simulink model "PID_Controller_referenceModel"  (R2021b)
settings: Solver=FixedStepDiscrete  StartTime=0.0  StopTime=10.0  FixedStep=Ts  RelTol=1e-3
PreLoadFcn:
  | %load('Parameters.mat')
values from neighbouring files (symbols this model uses):
  Kd = 1    [Parameters.mat]
  Ki = 1    [Parameters.mat]
  Kp = 1    [Parameters.mat]
  Ts = 0.01    [Parameters.mat]
settings Model: Creator=vigne  LastModifiedBy=vigne
settings DataIOCC: SaveOutput=off  SaveTime=off
settings OptimizationCC: DefaultParameterBehavior=Inlined  EnhancedBackFolding=on  PassReuseOutputArgsAs=Individual arguments  ZeroExternalMemoryAtStartup=off  ZeroInternalMemoryAtStartup=off  OptimizeBlockOrder=speed  DifferentSizesBufferReuse=on  OptimizationCustomize=off  EfficientTunableParamExpr=on
settings DebuggingCC: ParameterTunabilityLossMsg=error
settings SFSimCC: MATLABDynamicMemAlloc=off
settings RTWCC: Description=Embedded Coder  SystemTargetFile=ert.tlc  GenCodeOnly=on  TemplateMakefile=ert_default_tmf
settings CodeAppCC: ForceParamTrailComments=on  IgnoreCustomStorageClasses=off  OperatorAnnotations=on  SimulinkDataObjDesc=on  SFDataObjDesc=on  InsertBlockDesc=on
settings ERTTargetCC: TargetLangStandard=C99 (ISO)  GenerateSampleERTMain=on  InlinedParameterPlacement=NonHierarchical  ERTCustomFileTemplate=example_file_process.tlc

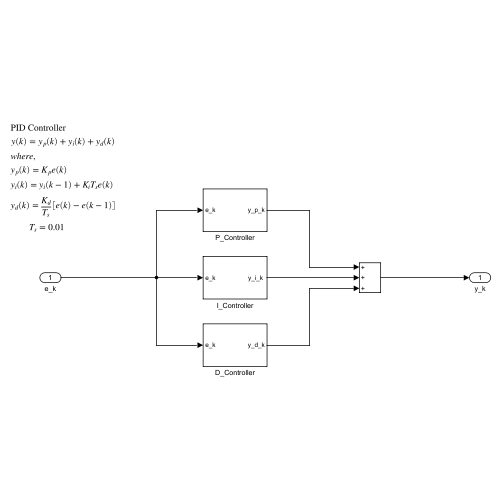
[thumbnail: Simulink's stored preview of the top-level diagram]
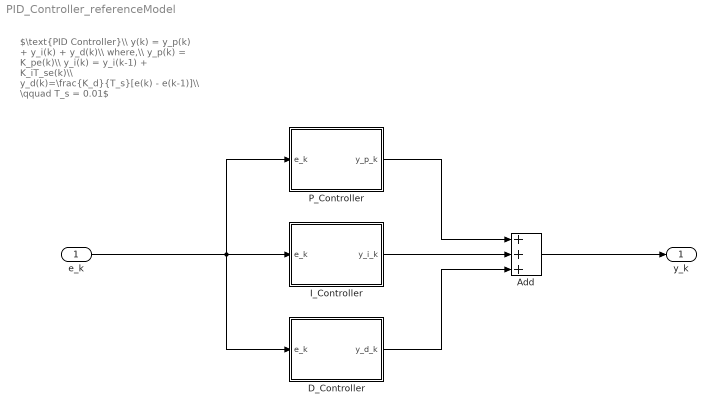
== system PID_Controller_referenceModel ==
  note: $\text{PID Controller}\\ y(k) = y_p(k) + y_i(k) + y_d(k)\\ where,\\ y_p(k) = K_pe(k)\\ y_i(k) = y_i(k-1) + K_iT_se(k)\\ y_d(k)=\frac{K_d}{T_s}[e(k) - e(k-1)]\\ \qquad T_s = 0.01$
  e_k : Inport  OutDataTypeStr=double  PortDimensions=1  SampleTime=Ts
  Add : Sum  Inputs=+++
  D_Controller : Subsystem
  I_Controller : Subsystem
  P_Controller : Subsystem
  y_k : Outport  OutDataTypeStr=double  PortDimensions=1  SampleTime=Ts
  wires:
  D_Controller/1(y_d_k) -> Add/3
  Add/1 -> y_k/1
  e_k/1 -> I_Controller/1(e_k), D_Controller/1(e_k), P_Controller/1(e_k)
  I_Controller/1("y_i_k ") -> Add/2
  P_Controller/1(y_p_k) -> Add/1

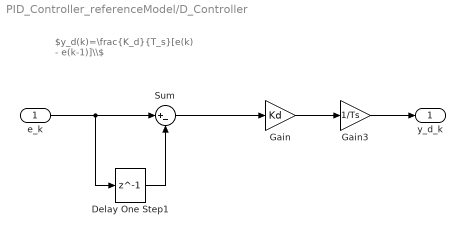
== system PID_Controller_referenceModel/D_Controller ==
  note: $y_d(k)=\frac{K_d}{T_s}[e(k) - e(k-1)]\\$
  e_k : Inport
  Delay One Step1 : Delay  DelayLength=1
  Gain : Gain  Gain=Kd
  Gain3 : Gain  Gain=1/Ts
  Sum : Sum  Inputs=|+-
  y_d_k : Outport
  wires:
  Gain/1 -> Gain3/1
  e_k/1 -> Delay One Step1/1, Sum/1
  Gain3/1 -> y_d_k/1
  Delay One Step1/1 -> Sum/2
  Sum/1 -> Gain/1

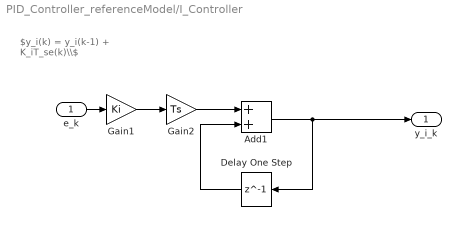
== system PID_Controller_referenceModel/I_Controller ==
  note: $y_i(k) = y_i(k-1) + K_iT_se(k)\\$
  e_k : Inport
  Add1 : Sum
  Delay One Step : Delay  DelayLength=1
  Gain1 : Gain  Gain=Ki
  Gain2 : Gain  Gain=Ts
  "y_i_k " : Outport
  wires:
  Delay One Step/1 -> Add1/2
  Gain1/1 -> Gain2/1
  Add1/1 -> Delay One Step/1, "y_i_k "/1
  Gain2/1 -> Add1/1
  e_k/1 -> Gain1/1

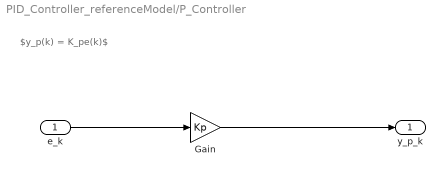
== system PID_Controller_referenceModel/P_Controller ==
  note: $y_p(k) = K_pe(k)$
  e_k : Inport
  Gain : Gain  Gain=Kp
  y_p_k : Outport
  wires:
  e_k/1 -> Gain/1
  Gain/1 -> y_p_k/1
